simulink model "airport_smo"  (R2025b)
settings: Solver=VariableStepAuto  StartTime=0.0  StopTime=100  RelTol=1e-3
undefined symbols (not defined in the file): m, n
settings Model: Creator=pavel  LastModifiedBy=pavel
settings SolverCC: AlgebraicLoopSolver=TrustRegion
settings DataIOCC: SaveOutput=off  SaveTime=off
settings DebuggingCC: UnconnectedInputMsg=warning  UnconnectedOutputMsg=warning  UnconnectedLineMsg=warning  ArithmeticOperatorsInVariantConditions=warning
settings ModelReferenceCC: EnableRefExpFcnMdlSchedulingChecks=on
settings SFSimCC: SimUseLocalCustomCode=off  CustomCodeUndefinedFunction=UseInterfaceOnly
settings RTWCC: RTWUseLocalCustomCode=off  GPUComputeCapability=3.5
settings CodeAppCC: StateflowObjectComments=on

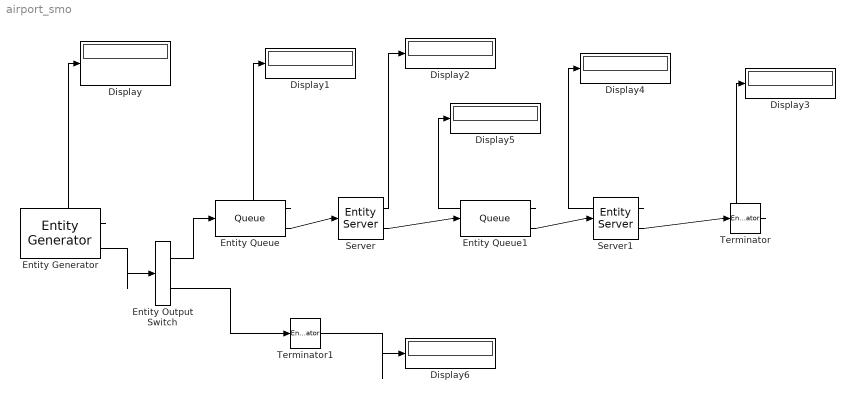
== system airport_smo ==
  " Server" : EntityServer  InputPortMessageModes=m  OutputPortMessageModes=n,m  Capacity=1  ServiceTimeValue=3  NumberEntitiesDeparted=on
      settings: OutputPortMap=o0,o9
  " Server1" : EntityServer  InputPortMessageModes=m  OutputPortMessageModes=n,m  Capacity=3  ServiceTimeValue=50  NumberEntitiesDeparted=on
      settings: OutputPortMap=o0,o9
  Display{,1..6} (7 alike) : Display
  Entity Output Switch : EntityOutputSwitch  InputPortMessageModes=m  OutputPortMessageModes=m,m  SwitchAttributeName=Attribute1
  Entity Generator : EntityGenerator  OutputPortMessageModes=n,m  Period=0.2  NumberEntitiesDeparted=on  EntityType=Structured  EntityTypeName=Entity
      settings: OutputPortMap=o0,o3
  Entity Queue : Queue  InputPortMessageModes=m  OutputPortMessageModes=n,m  Capacity=30  NumberEntitiesInBlock=on
      settings: OutputPortMap=o1,o5
  Entity Queue1 : Queue  InputPortMessageModes=m  OutputPortMessageModes=n,m  Capacity=10  NumberEntitiesInBlock=on
      settings: OutputPortMap=o1,o5
  Terminator : EntityTerminator  InputPortMessageModes=m  NumberEntitiesArrived=on
      settings: OutputPortMap=o0
  Terminator1 : EntityTerminator  InputPortMessageModes=m  NumberEntitiesArrived=on
      settings: OutputPortMap=o0
  wires:
  " Server"/1 -> Display2/1
  Entity Generator/1 -> Display/1
  Entity Queue/2 -> " Server"/1
  Terminator/1 -> Display3/1
  Entity Queue1/2 -> " Server1"/1
  " Server"/2 -> Entity Queue1/1
  " Server1"/2 -> Terminator/1
  " Server1"/1 -> Display4/1
  Entity Queue/1 -> Display1/1
  Entity Queue1/1 -> Display5/1
  Entity Generator/2 -> Entity Output Switch/1
  Entity Output Switch/1 -> Entity Queue/1
  Entity Output Switch/2 -> Terminator1/1
  Terminator1/1 -> Display6/1
